simulink model "observer"  (R2018b)
settings: Solver=VariableStepAuto  StartTime=0.0  StopTime=2  RelTol=1e-3
undefined symbols (not defined in the file): A, B, C, D, F1, F2, k, K_lqr, Lo, R, To
settings Model: Creator=Amin  LastModifiedBy=tayeb
settings SFSimCC: SimUseLocalCustomCode=off
settings RTWCC: RTWUseLocalCustomCode=off
settings CodeAppCC: StateflowObjectComments=on

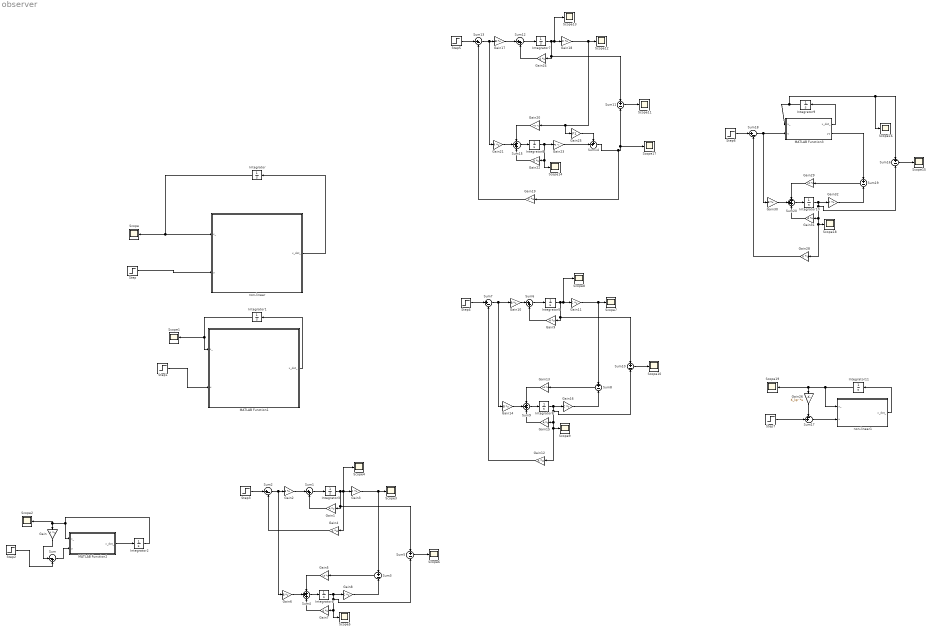
== system observer ==
  Gain{,4,12,19,28} (5 alike) : Gain  Gain=k  Multiplication=Matrix(K*u)
  Gain{1,7,9,15,24,31} (6 alike) : Gain  Gain=A  Multiplication=Matrix(K*u)
  Gain{2,6,10,14,17,30} (6 alike) : Gain  Gain=B  Multiplication=Matrix(K*u)
  Gain{3,8,11,16,18,32} (6 alike) : Gain  Gain=C  Multiplication=Matrix(K*u)
  Gain13 : Gain  Gain=Lo  Multiplication=Matrix(K*u)
  Gain20 : Gain  Gain=To  Multiplication=Matrix(K*u)
  Gain21 : Gain  Gain=R  Multiplication=Matrix(K*u)
  Gain22 : Gain  Gain=D  Multiplication=Matrix(K*u)
  Gain23 : Gain  Gain=F2  Multiplication=Matrix(K*u)
  Gain25 : Gain  Gain=F1
  Gain26 : Gain  Gain=K_lqr  Multiplication=Matrix(K*u)
  Gain29 : Gain  Gain=Lo  Multiplication=Matrix(K*u)
  Gain5 : Gain  Gain=Lo  Multiplication=Matrix(K*u)
  Integrator : Integrator  InitialCondition=[0 0 0.5 0]
  Integrator1 : Integrator  InitialCondition=[0 0 0.5 0]
  Integrator10 : Integrator  InitialCondition=[0 0 0 0]
  Integrator11 : Integrator  InitialCondition=[0 0 0.5 0]
  Integrator2 : Integrator  InitialCondition=[0.1 0 0.5 0]
  Integrator3 : Integrator  InitialCondition=[0.2 0 0 0]
  Integrator4 : Integrator  InitialCondition=[0 0 0 0]
  Integrator5 : Integrator  InitialCondition=[0.2 0 0 0]
  Integrator6 : Integrator  InitialCondition=[0 0 0 0]
  Integrator7 : Integrator  InitialCondition=[0.2 0 0 0]
  Integrator8 : Integrator  InitialCondition=[0 0 0]
  Integrator9 : Integrator  InitialCondition=[0.1 0 0 0]
  MATLAB Function1 : MATLAB Function  TreatAsAtomicUnit=on
  MATLAB Function2 : MATLAB Function  TreatAsAtomicUnit=on
  MATLAB Function3 : MATLAB Function  TreatAsAtomicUnit=on
  Scope{,1..19} (20 alike) : Scope
  Step : Step  After=3  SampleTime=0
  Step1 : Step  After=3  SampleTime=0
  Step{2..7} (6 alike) : Step  After=0  SampleTime=0
  Sum : Sum  Inputs=|-+
  Sum1 : Sum  Inputs=|++
  Sum{3,5,8,10..11,16,19} (7 alike) : Sum  Inputs=+|-
  Sum12 : Sum  Inputs=|++
  Sum{2,7,13,18} (4 alike) : Sum  Inputs=|+-
  Sum14 : Sum  Inputs=++|
  Sum{4,9,15,20} (4 alike) : Sum  Inputs=+++
  Sum17 : Sum  Inputs=-+|
  Sum6 : Sum  Inputs=|++
  non-linear : MATLAB Function  TreatAsAtomicUnit=on
  non-linear1 : MATLAB Function  TreatAsAtomicUnit=on
  wires:
  non-linear/1(x_dot_) -> Integrator/1
  Integrator/1 -> Scope/1, non-linear/1(x_)
  Step/1 -> non-linear/2(u)
  Step1/1 -> MATLAB Function1/2(u)
  Integrator1/1 -> Scope1/1, MATLAB Function1/1(x_)
  MATLAB Function1/1(x_dot_) -> Integrator1/1
  Integrator2/1 -> MATLAB Function2/1(x_), Scope2/1, Gain/1
  MATLAB Function2/1(x_dot_) -> Integrator2/1
  Gain/1 -> Sum/1
  Step2/1 -> Sum/2
  Sum/1 -> MATLAB Function2/2(u)
  Gain2/1 -> Sum1/1
  Gain3/1 -> Sum3/1, Scope3/1
  Sum1/1 -> Integrator3/1
  Gain1/1 -> Sum1/2
  Integrator3/1 -> Sum5/1, Gain1/1, Gain4/1, Scope4/1, Gain3/1
  Sum2/1 -> Gain6/1, Gain2/1
  Gain4/1 -> Sum2/2
  Step3/1 -> Sum2/1
  Sum3/1 -> Gain5/1
  Sum4/1 -> Integrator4/1
  Gain5/1 -> Sum4/1
  Gain6/1 -> Sum4/2
  Gain7/1 -> Sum4/3
  Integrator4/1 -> Gain8/1, Sum5/2, Scope5/1, Gain7/1
  Gain8/1 -> Sum3/2
  Sum5/1 -> Scope6/1
  Gain9/1 -> Sum6/2
  Sum6/1 -> Integrator5/1
  Gain10/1 -> Sum6/1
  Gain16/1 -> Sum8/2
  Gain13/1 -> Sum9/1
  Integrator6/1 -> Gain16/1, Sum10/2, Gain12/1, Scope9/1, Gain15/1
  Step4/1 -> Sum7/1
  Sum9/1 -> Integrator6/1
  Gain11/1 -> Sum8/1, Scope7/1
  Gain15/1 -> Sum9/3
  Integrator5/1 -> Sum10/1, Gain9/1, Scope8/1, Gain11/1
  Gain14/1 -> Sum9/2
  Sum7/1 -> Gain14/1, Gain10/1
  Sum10/1 -> Scope10/1
  Sum8/1 -> Gain13/1
  Gain12/1 -> Sum7/2
  Sum12/1 -> Integrator7/1
  Step5/1 -> Sum13/1
  Integrator7/1 -> Gain24/1, Sum11/1, Scope13/1, Gain18/1
  Gain21/1 -> Sum15/2
  Integrator8/1 -> Gain23/1, Scope14/1, Gain22/1
  Sum15/1 -> Integrator8/1
  Sum13/1 -> Gain21/1, Gain17/1
  Gain22/1 -> Sum15/3
  Sum11/1 -> Scope11/1
  Gain19/1 -> Sum13/2
  Gain17/1 -> Sum12/1
  Gain20/1 -> Sum15/1
  Gain24/1 -> Sum12/2
  Gain18/1 -> Gain25/1, Gain20/1, Scope12/1
  Gain23/1 -> Sum14/2
  Gain25/1 -> Sum14/1
  Sum14/1 -> Gain19/1, Sum11/2, Scope17/1
  Gain28/1 -> Sum18/2
  Sum16/1 -> Scope15/1
  Sum19/1 -> Gain29/1
  Step6/1 -> Sum18/1
  Gain29/1 -> Sum20/1
  Gain32/1 -> Sum19/2
  Sum20/1 -> Integrator10/1
  Integrator10/1 -> Gain32/1, Sum16/2, Gain28/1, Scope18/1, Gain31/1
  Sum18/1 -> MATLAB Function3/2(u), Gain30/1
  Gain31/1 -> Sum20/3
  Gain30/1 -> Sum20/2
  Integrator9/1 -> Sum16/1, Scope16/1, MATLAB Function3/1(x_)
  MATLAB Function3/1(x_dot_) -> Integrator9/1
  MATLAB Function3/2(yy) -> Sum19/1
  non-linear1/1(x_dot_) -> Integrator11/1
  Integrator11/1 -> Scope19/1, Gain26/1, non-linear1/1(x_)
  Sum17/1 -> non-linear1/2(u)
  Gain26/1 -> Sum17/1
  Step7/1 -> Sum17/2

== matlab function observer/MATLAB Function1 ==
  data: x_ input; x_dot_ output; u input
function x_dot_  = fcn(x_ , u )

x = x_(1);
phi = x_(2);
x_dot = x_(3);
phi_dot = x_(4);
v = u;

MB = 0.77 ;
L = 0.128 ;
Mb = 0.01 ;
Rb = 0.026 ; 
IBx = 0.003677;
IBy = 0.003927 ;
Ib = 0;
n = (-30/52)*(-20/12);
IM = 2*10^(-5);
Meu_Bb = 0.0022 ;
Meu_Bg = 0;
g = 10 ;

% Servo_Motor 
Kt = 0.317 ;
Kb = 0.468 ; 
Rm = 6.69 ; 

Dx = IBx*IM + IM*Ib - 2*IM*Ib*n + IBx*Ib*n*n + IM*Ib*n*n + IM*L*L*MB + IM*MB*Rb*Rb + IM*Mb*Rb*Rb + Ib*L*L*MB*n*n + IBx*MB*n*n*Rb*Rb + IM*MB*n*n*Rb*Rb + IBx*Mb*n*n*Rb*Rb + IM*Mb*n*n*Rb*Rb + 2*IM*L*MB*Rb - 2*IM*MB*n*Rb*Rb - 2*IM*Mb*n*Rb*Rb + L*L*MB*Mb*n*n*Rb*Rb - 2*IM*L*MB*n*Rb ; 
Dy = IBy*IM + IM*Ib - 2*IM*Ib*n + IBy*Ib*n*n + IM*Ib*n*n + IM*L*L*MB + IM*MB*Rb*Rb + IM*Mb*Rb*Rb + Ib*L*L*MB*n*n + IBy*MB*n*n*Rb*Rb + IM*MB*n*n*Rb*Rb + IBy*Mb*n*n*Rb*Rb + IM*Mb*n*n*Rb*Rb + 2*IM*L*MB*Rb - 2*IM*MB*n*Rb*Rb - 2*IM*Mb*n*Rb*Rb + L*L*MB*Mb*n*n*Rb*Rb - 2*IM*L*MB*n*Rb ; 


Ax_31 = g*L*MB*(IM + Ib*n*n + MB*n*n*Rb*Rb + Mb*n*n*Rb*Rb)/Dx ; 
Ax_41 = -g*L*MB*(IM + Ib*n + MB*n*Rb*Rb + Mb*n*Rb*Rb + L*MB*n*Rb)/Dx ;
Ax_33 = -Meu_Bg*(IM + Ib*n*n  + MB*n*n*Rb*Rb + Mb*n*n*Rb*Rb)/Dx ;
Ax_43 = Meu_Bg*(IM + Ib*n + MB*n*Rb*Rb + Mb*n*n*Rb*Rb + L*MB*n*Rb)/Dx ;
Ax_34 = (Meu_Bb + ((Kb*Kt)/Rm)*(IM + Ib*n + MB*n*Rb*Rb + Mb*n*Rb*Rb + L*MB*n*Rb))/Dx ;
Ax_44 = -(Meu_Bb + ((Kb*Kt)/Rm)*(IBx + IM + Ib + L*L*MB +  MB*Rb*Rb + Mb*Rb*Rb + 2*L*MB*Rb))/Dx ;

Ay_44 = -(Meu_Bb + ((Kb*Kt)/Rm)*(IBy + IM + Ib + L*L*MB +  MB*Rb*Rb + Mb*Rb*Rb + 2*L*MB*Rb))/Dy ;
Ay_33 = -Meu_Bg*(IM + Ib*n*n  + MB*n*n*Rb*Rb + Mb*n*n*Rb*Rb)/Dy ;
Ay_34 = (Meu_Bb + ((Kb*Kt)/Rm)*(IM + Ib*n + MB*n*Rb*Rb + Mb*n*Rb*Rb + L*MB*n*Rb))/Dy ;
Ay_43 = Meu_Bg*(IM + Ib*n + MB*n*Rb*Rb + Mb*n*n*Rb*Rb + L*MB*n*Rb)/Dy ;
Ay_31 = g*L*MB*(IM + Ib*n*n + MB*n*n*Rb*Rb + Mb*n*n*Rb*Rb)/Dy ; 
Ay_41 = -g*L*MB*(IM + Ib*n + MB*n*Rb*Rb + Mb*n*Rb*Rb + L*MB*n*Rb)/Dy ;


Bx_31 = -Kt*(IM + Ib*n + MB*n*Rb*Rb + Mb*n*Rb*Rb + L*MB*n*Rb)/(Dx*Rm) ;
Bx_41 = Kt*(IBx + IM + Ib + L*L*MB +  MB*Rb*Rb + Mb*Rb*Rb + 2*L*MB*Rb)/(Dx*Rm) ; 

By_31 = -Kt*(IM + Ib*n + MB*n*Rb*Rb + Mb*n*Rb*Rb + L*MB*n*Rb)/(Dy*Rm) ;
By_41 = Kt*(IBy + IM + Ib + L*L*MB +  MB*Rb*Rb + Mb*Rb*Rb + 2*L*MB*Rb)/(Dy*Rm) ; 



A = [ 0 0 1 0 ; 0 0 0 1; Ax_31 0 Ax_33 Ax_34 ; Ax_41 0 Ax_43 Ax_44]
B = [ 0  ; 0  ; Bx_31  ; Bx_41  ]

C = [ 0 1 0 0   ];
D = 0 ;

x_dot_ = A*x_ + B*u;


end

== matlab function observer/non-linear ==
  data: x_ input; x_dot_ output; u input
function x_dot_  = fcn(x_ , u )

x = x_(1);
phi = x_(2);
x_dot = x_(3);
phi_dot = x_(4);
v = u;
% parameters 
MB = 0.77 ;
L = 0.128 ;
Mb = 0.01 ;
Rb = 0.026 ; 
IBx = 0.003677;
IBy = 0.003927 ;
Ib = 0;
n = (-30/52)*(-20/12);
IM = 2*10^(-5);
Meu_Bb = 0.0022 ;
Meu_Bg = 0;
g = 10 ;

% Servo_Motor 
Kt = 0.317 ;
Kb = 0.468 ; 
Rm = 6.69 ; 


Mx_11 = IBx + IM + Ib + L*L*MB + MB*Rb*Rb + Mb*Rb*Rb + 2*L*MB*Rb*cos(x);
Mx_12 = IM + Ib*n + MB*n*Rb*Rb + Mb*n*Rb*Rb + L*MB*n*Rb*cos(x);
Mx_21 = IM + Ib*n + MB*n*Rb*Rb + Mb*n*Rb*Rb + L*MB*n*Rb*cos(x);
Mx_22 = IM + Ib*n*n + MB*n*n*Rb*Rb + Mb*n*n*Rb*Rb ; 

%Mass Function 
M =[Mx_11 , Mx_12 ; Mx_21 , Mx_22] ;

% 
Rx = [ -L*MB*Rb*sin(x)*(x_dot)*(x_dot) - g*L*MB*sin(x) ; -L*MB*n*Rb*x_dot*x_dot*sin(x)] ;

% Force matrix
Fx = [ -Meu_Bg*x_dot ; Kt*v/Rm - Meu_Bb*phi_dot - (Kb*Kt*phi_dot)/Rm ] ;

% output 
x_d = x_dot ;
phi_d = phi_dot ; 

aa =inv(M)*(Fx - Rx);
x_double_d = aa(1);
phi_double_d = aa(2); 

x_dot_ = [x_d , phi_d , x_double_d , phi_double_d ];
end

== matlab function observer/MATLAB Function2 ==
  data: x_ input; x_dot_ output; u input
function x_dot_  = fcn(x_ , u )

x = x_(1);
phi = x_(2);
x_dot = x_(3);
phi_dot = x_(4);
v = u;

MB = 0.77 ;
L = 0.128 ;
Mb = 0.01 ;
Rb = 0.026 ; 
IBx = 0.003677;
IBy = 0.003927 ;
Ib = 0;
n = (-30/52)*(-20/12);
IM = 2*10^(-5);
Meu_Bb = 0.0022 ;
Meu_Bg = 0;
g = 10 ;

% Servo_Motor 
Kt = 0.317 ;
Kb = 0.468 ; 
Rm = 6.69 ; 

Dx = IBx*IM + IM*Ib - 2*IM*Ib*n + IBx*Ib*n*n + IM*Ib*n*n + IM*L*L*MB + IM*MB*Rb*Rb + IM*Mb*Rb*Rb + Ib*L*L*MB*n*n + IBx*MB*n*n*Rb*Rb + IM*MB*n*n*Rb*Rb + IBx*Mb*n*n*Rb*Rb + IM*Mb*n*n*Rb*Rb + 2*IM*L*MB*Rb - 2*IM*MB*n*Rb*Rb - 2*IM*Mb*n*Rb*Rb + L*L*MB*Mb*n*n*Rb*Rb - 2*IM*L*MB*n*Rb ; 
Dy = IBy*IM + IM*Ib - 2*IM*Ib*n + IBy*Ib*n*n + IM*Ib*n*n + IM*L*L*MB + IM*MB*Rb*Rb + IM*Mb*Rb*Rb + Ib*L*L*MB*n*n + IBy*MB*n*n*Rb*Rb + IM*MB*n*n*Rb*Rb + IBy*Mb*n*n*Rb*Rb + IM*Mb*n*n*Rb*Rb + 2*IM*L*MB*Rb - 2*IM*MB*n*Rb*Rb - 2*IM*Mb*n*Rb*Rb + L*L*MB*Mb*n*n*Rb*Rb - 2*IM*L*MB*n*Rb ; 


Ax_31 = g*L*MB*(IM + Ib*n*n + MB*n*n*Rb*Rb + Mb*n*n*Rb*Rb)/Dx ; 
Ax_41 = -g*L*MB*(IM + Ib*n + MB*n*Rb*Rb + Mb*n*Rb*Rb + L*MB*n*Rb)/Dx ;
Ax_33 = -Meu_Bg*(IM + Ib*n*n  + MB*n*n*Rb*Rb + Mb*n*n*Rb*Rb)/Dx ;
Ax_43 = Meu_Bg*(IM + Ib*n + MB*n*Rb*Rb + Mb*n*n*Rb*Rb + L*MB*n*Rb)/Dx ;
Ax_34 = (Meu_Bb + ((Kb*Kt)/Rm)*(IM + Ib*n + MB*n*Rb*Rb + Mb*n*Rb*Rb + L*MB*n*Rb))/Dx ;
Ax_44 = -(Meu_Bb + ((Kb*Kt)/Rm)*(IBx + IM + Ib + L*L*MB +  MB*Rb*Rb + Mb*Rb*Rb + 2*L*MB*Rb))/Dx ;

Ay_44 = -(Meu_Bb + ((Kb*Kt)/Rm)*(IBy + IM + Ib + L*L*MB +  MB*Rb*Rb + Mb*Rb*Rb + 2*L*MB*Rb))/Dy ;
Ay_33 = -Meu_Bg*(IM + Ib*n*n  + MB*n*n*Rb*Rb + Mb*n*n*Rb*Rb)/Dy ;
Ay_34 = (Meu_Bb + ((Kb*Kt)/Rm)*(IM + Ib*n + MB*n*Rb*Rb + Mb*n*Rb*Rb + L*MB*n*Rb))/Dy ;
Ay_43 = Meu_Bg*(IM + Ib*n + MB*n*Rb*Rb + Mb*n*n*Rb*Rb + L*MB*n*Rb)/Dy ;
Ay_31 = g*L*MB*(IM + Ib*n*n + MB*n*n*Rb*Rb + Mb*n*n*Rb*Rb)/Dy ; 
Ay_41 = -g*L*MB*(IM + Ib*n + MB*n*Rb*Rb + Mb*n*Rb*Rb + L*MB*n*Rb)/Dy ;


Bx_31 = -Kt*(IM + Ib*n + MB*n*Rb*Rb + Mb*n*Rb*Rb + L*MB*n*Rb)/(Dx*Rm) ;
Bx_41 = Kt*(IBx + IM + Ib + L*L*MB +  MB*Rb*Rb + Mb*Rb*Rb + 2*L*MB*Rb)/(Dx*Rm) ; 

By_31 = -Kt*(IM + Ib*n + MB*n*Rb*Rb + Mb*n*Rb*Rb + L*MB*n*Rb)/(Dy*Rm) ;
By_41 = Kt*(IBy + IM + Ib + L*L*MB +  MB*Rb*Rb + Mb*Rb*Rb + 2*L*MB*Rb)/(Dy*Rm) ; 



A = [ 0 0 1 0 ; 0 0 0 1; Ax_31 0 Ax_33 Ax_34 ; Ax_41 0 Ax_43 Ax_44]
B = [ 0  ; 0  ; Bx_31  ; Bx_41  ]

C = [ 0 1 0 0   ];
D = 0 ;

x_dot_ = A*x_ + B*u;


end

== matlab function observer/MATLAB Function3 ==
  data: x_ input; x_dot_ output; u input; yy output
function [x_dot_ , yy] = fcn(x_ , u )

x = x_(1);
phi = x_(2);
x_dot = x_(3);
phi_dot = x_(4);
v = u;

MB = 0.77 ;
L = 0.128 ;
Mb = 0.01 ;
Rb = 0.026 ; 
IBx = 0.003677;
IBy = 0.003927 ;
Ib = 0;
n = (-30/52)*(-20/12);
IM = 2*10^(-5);
Meu_Bb = 0.0022 ;
Meu_Bg = 0;
g = 10 ;

% Servo_Motor 
Kt = 0.317 ;
Kb = 0.468 ; 
Rm = 6.69 ; 

Dx = IBx*IM + IM*Ib - 2*IM*Ib*n + IBx*Ib*n*n + IM*Ib*n*n + IM*L*L*MB + IM*MB*Rb*Rb + IM*Mb*Rb*Rb + Ib*L*L*MB*n*n + IBx*MB*n*n*Rb*Rb + IM*MB*n*n*Rb*Rb + IBx*Mb*n*n*Rb*Rb + IM*Mb*n*n*Rb*Rb + 2*IM*L*MB*Rb - 2*IM*MB*n*Rb*Rb - 2*IM*Mb*n*Rb*Rb + L*L*MB*Mb*n*n*Rb*Rb - 2*IM*L*MB*n*Rb ; 
Dy = IBy*IM + IM*Ib - 2*IM*Ib*n + IBy*Ib*n*n + IM*Ib*n*n + IM*L*L*MB + IM*MB*Rb*Rb + IM*Mb*Rb*Rb + Ib*L*L*MB*n*n + IBy*MB*n*n*Rb*Rb + IM*MB*n*n*Rb*Rb + IBy*Mb*n*n*Rb*Rb + IM*Mb*n*n*Rb*Rb + 2*IM*L*MB*Rb - 2*IM*MB*n*Rb*Rb - 2*IM*Mb*n*Rb*Rb + L*L*MB*Mb*n*n*Rb*Rb - 2*IM*L*MB*n*Rb ; 


Ax_31 = g*L*MB*(IM + Ib*n*n + MB*n*n*Rb*Rb + Mb*n*n*Rb*Rb)/Dx ; 
Ax_41 = -g*L*MB*(IM + Ib*n + MB*n*Rb*Rb + Mb*n*Rb*Rb + L*MB*n*Rb)/Dx ;
Ax_33 = -Meu_Bg*(IM + Ib*n*n  + MB*n*n*Rb*Rb + Mb*n*n*Rb*Rb)/Dx ;
Ax_43 = Meu_Bg*(IM + Ib*n + MB*n*Rb*Rb + Mb*n*n*Rb*Rb + L*MB*n*Rb)/Dx ;
Ax_34 = (Meu_Bb + ((Kb*Kt)/Rm)*(IM + Ib*n + MB*n*Rb*Rb + Mb*n*Rb*Rb + L*MB*n*Rb))/Dx ;
Ax_44 = -(Meu_Bb + ((Kb*Kt)/Rm)*(IBx + IM + Ib + L*L*MB +  MB*Rb*Rb + Mb*Rb*Rb + 2*L*MB*Rb))/Dx ;

Ay_44 = -(Meu_Bb + ((Kb*Kt)/Rm)*(IBy + IM + Ib + L*L*MB +  MB*Rb*Rb + Mb*Rb*Rb + 2*L*MB*Rb))/Dy ;
Ay_33 = -Meu_Bg*(IM + Ib*n*n  + MB*n*n*Rb*Rb + Mb*n*n*Rb*Rb)/Dy ;
Ay_34 = (Meu_Bb + ((Kb*Kt)/Rm)*(IM + Ib*n + MB*n*Rb*Rb + Mb*n*Rb*Rb + L*MB*n*Rb))/Dy ;
Ay_43 = Meu_Bg*(IM + Ib*n + MB*n*Rb*Rb + Mb*n*n*Rb*Rb + L*MB*n*Rb)/Dy ;
Ay_31 = g*L*MB*(IM + Ib*n*n + MB*n*n*Rb*Rb + Mb*n*n*Rb*Rb)/Dy ; 
Ay_41 = -g*L*MB*(IM + Ib*n + MB*n*Rb*Rb + Mb*n*Rb*Rb + L*MB*n*Rb)/Dy ;


Bx_31 = -Kt*(IM + Ib*n + MB*n*Rb*Rb + Mb*n*Rb*Rb + L*MB*n*Rb)/(Dx*Rm) ;
Bx_41 = Kt*(IBx + IM + Ib + L*L*MB +  MB*Rb*Rb + Mb*Rb*Rb + 2*L*MB*Rb)/(Dx*Rm) ; 

By_31 = -Kt*(IM + Ib*n + MB*n*Rb*Rb + Mb*n*Rb*Rb + L*MB*n*Rb)/(Dy*Rm) ;
By_41 = Kt*(IBy + IM + Ib + L*L*MB +  MB*Rb*Rb + Mb*Rb*Rb + 2*L*MB*Rb)/(Dy*Rm) ; 



A = [ 0 0 1 0 ; 0 0 0 1; Ax_31 0 Ax_33 Ax_34 ; Ax_41 0 Ax_43 Ax_44]
B = [ 0  ; 0  ; Bx_31  ; Bx_41  ]

C = [ 0 1 0 0   ];
D = 0 ;

x_dot_ = A*x_ + B*u;
yy = C * x_;

end

== matlab function observer/non-linear1 ==
  data: x_ input; x_dot_ output; u input
function x_dot_  = fcn(x_ , u )

x = x_(1);
phi = x_(2);
x_dot = x_(3);
phi_dot = x_(4);
v = u;
% parameters 
MB = 0.77 ;
L = 0.128 ;
Mb = 0.01 ;
Rb = 0.026 ; 
IBx = 0.003677;
IBy = 0.003927 ;
Ib = 0;
n = (-30/52)*(-20/12);
IM = 2*10^(-5);
Meu_Bb = 0.0022 ;
Meu_Bg = 0;
g = 10 ;

% Servo_Motor 
Kt = 0.317 ;
Kb = 0.468 ; 
Rm = 6.69 ; 


Mx_11 = IBx + IM + Ib + L*L*MB + MB*Rb*Rb + Mb*Rb*Rb + 2*L*MB*Rb*cos(x);
Mx_12 = IM + Ib*n + MB*n*Rb*Rb + Mb*n*Rb*Rb + L*MB*n*Rb*cos(x);
Mx_21 = IM + Ib*n + MB*n*Rb*Rb + Mb*n*Rb*Rb + L*MB*n*Rb*cos(x);
Mx_22 = IM + Ib*n*n + MB*n*n*Rb*Rb + Mb*n*n*Rb*Rb ; 

%Mass Function 
M =[Mx_11 , Mx_12 ; Mx_21 , Mx_22] ;

% 
Rx = [ -L*MB*Rb*sin(x)*(x_dot)*(x_dot) - g*L*MB*sin(x) ; -L*MB*n*Rb*x_dot*x_dot*sin(x)] ;

% Force matrix
Fx = [ -Meu_Bg*x_dot ; Kt*v/Rm - Meu_Bb*phi_dot - (Kb*Kt*phi_dot)/Rm ] ;

% output 
x_d = x_dot ;
phi_d = phi_dot ; 

aa =inv(M)*(Fx - Rx);
x_double_d = aa(1);
phi_double_d = aa(2); 

x_dot_ = [x_d , phi_d , x_double_d , phi_double_d ];
end
